simulink model "mapminmax_reverse1"  (R2017b)
settings: Solver=VariableStepAuto  StartTime=0.0  StopTime=10.0  RelTol=1e-3
undefined symbols (not defined in the file or in its folder): NNout
settings Model: Creator=awur978  LastModifiedBy=awur978

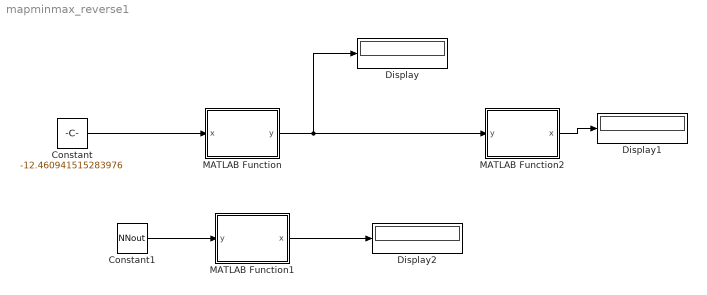
== system mapminmax_reverse1 ==
  Constant : Constant  Value=-12.460941515283976
  Constant1 : Constant  Value=NNout
  Display : Display
  Display1 : Display
  Display2 : Display
  MATLAB Function : MATLAB Function  TreatAsAtomicUnit=on
  MATLAB Function1 : MATLAB Function  TreatAsAtomicUnit=on
  MATLAB Function2 : MATLAB Function  TreatAsAtomicUnit=on
  wires:
  MATLAB Function/1(y) -> Display/1, MATLAB Function2/1(y)
  Constant/1 -> MATLAB Function/1(x)
  MATLAB Function2/1(x) -> Display1/1
  Constant1/1 -> MATLAB Function1/1(y)
  MATLAB Function1/1(x) -> Display2/1

== matlab function mapminmax_reverse1/MATLAB Function1 ==
  data: y input; x output
function x =mapminmax_reverse(y)
   ymax = 1;ymin=-1;xmin=-12.4609;xmax=7.0414;
    x=(((y*(xmax-xmin)) -( ymin*(xmax-xmin)))/(ymax-ymin))+xmin;
end

== matlab function mapminmax_reverse1/MATLAB Function ==
  data: x input; y output
function y =mapminmax_forward(x)
    ymax = 1;ymin=-1;xmin=-12.4609;xmax=7.0414;
    y = (ymax-ymin)*(x-xmin)/(xmax-xmin) + ymin;
end

== matlab function mapminmax_reverse1/MATLAB Function2 ==
  data: y input; x output
function x =mapminmax_reverse(y)
   ymax = 1;ymin=-1;xmin=-12.4609;xmax=7.0414;
    x=(((y*(xmax-xmin)) -( ymin*(xmax-xmin)))/(ymax-ymin))+xmin;
end
